simulink model "text"  (R2022a)
settings: Solver=FixedStepAuto  StartTime=0.0  StopTime=10.0  FixedStep=1e-3  RelTol=1e-3  EnableMultiTasking=on
undefined symbols (not defined in the file): A0, A1, D0, D1, PTB2, PTB3, PTC16, PTC17
libraries: etargetslib x16, frdmk64flib x6
settings Model: ExtModeTrigDuration=5  Creator=12791  LastModifiedBy=12791
settings OptimizationCC: EnhancedBackFolding=on  PassReuseOutputArgsAs=Individual arguments  ZeroExternalMemoryAtStartup=off  ZeroInternalMemoryAtStartup=off  MaxStackSize=64  OptimizeBlockOrder=speed  DifferentSizesBufferReuse=on  OptimizationCustomize=off  EfficientTunableParamExpr=on
settings DebuggingCC: ParameterTunabilityLossMsg=error
settings HardwareCC: ProdBitPerPointer=32  ProdBitPerSizeT=32  ProdBitPerPtrDiffT=32  ProdLargestAtomicInteger=Long  ProdLargestAtomicFloat=Double  ProdWordSize=32  ProdHWDeviceType=ARM Compatible->ARM Cortex
settings SFSimCC: MATLABDynamicMemAlloc=off
settings RTWCC: SystemTargetFile=ert.tlc  HardwareBoard=NXP FRDM-K64F  TLCOptions="-aInlineSetEventsForThisBaseRateFcn=TLC_FALSE -aSuppressMultiTaskScheduler=TLC_FALSE  -aRateBasedStepFcn=0"  TemplateMakefile=ert_default_tmf  Toolchain=GNU Tools for ARM Embedded Processors
settings CodeAppCC: ForceParamTrailComments=on  IgnoreCustomStorageClasses=off  OperatorAnnotations=on  SimulinkDataObjDesc=on  SFDataObjDesc=on  InsertBlockDesc=on
settings ERTTargetCC: ExtModeTransport=4  ExtModeMexFile=sendToCommService

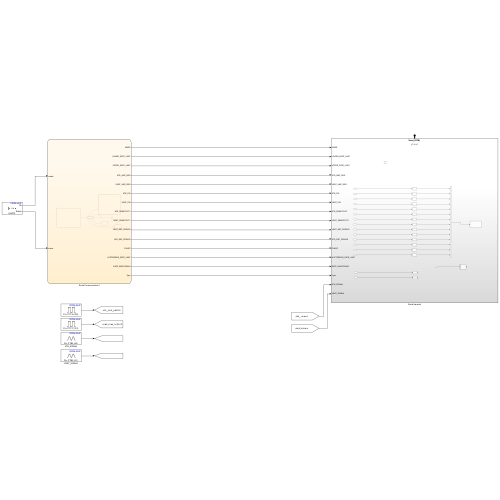
[thumbnail: Simulink's stored preview of the top-level diagram]
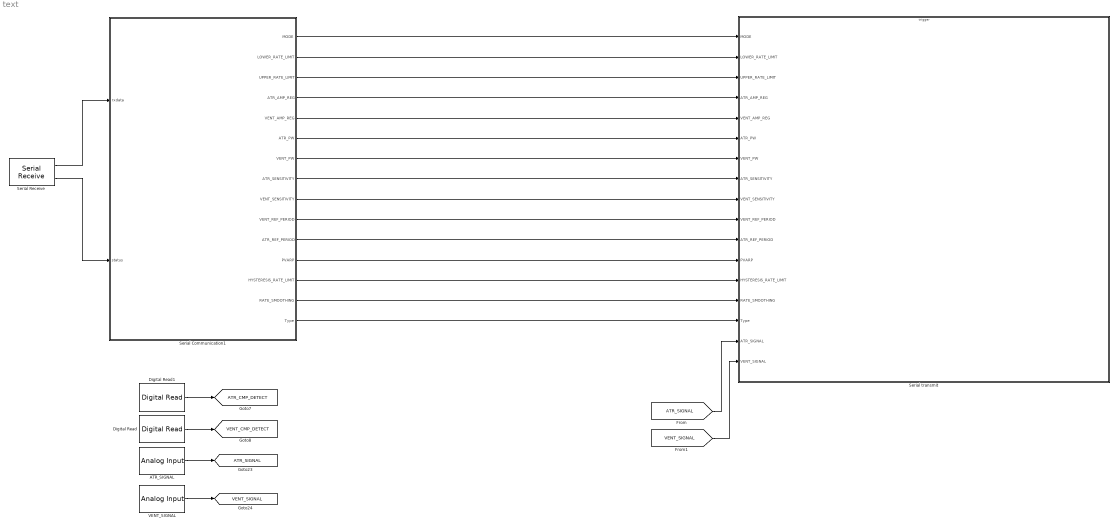
== system text ==
  ATR_SIGNAL : frdmk64flib/Analog Input  Whichpin=PTB2 (A0)  SampleTime=-1
  Digital Read : frdmk64flib/Digital Read  Whichpin=PTC17 (D1)  SampleTime=-1
  Digital Read1 : frdmk64flib/Digital Read  Whichpin=PTC16 (D0)  SampleTime=-1
  Serial Communication1 : Stateflow chart  TreatAsAtomicUnit=on
      settings: PortSchema="{\"entries\":[{\"content\":{\"sides\":[{\"content\":{\"connectorIds\":[\"In1\",\"In2\"]},\"type\":\"ConnectorPlacement.EquallySpacedRectSide\",\"uuid\":\"901574a5-7e09-4852-8827-baac8e876273\"},{\"content\":{\"connectorIds\":[\"Out1\",\"Out2\",\"Out3\",\"Out4\",\"Out12\",\"Out5\",\"Out13\",\"Out14\",\"Out10\",\"Out6\",\"Out11\",\"Out7\",\"Out9\",\"Out8\",\"Out15\"],\"side\":\"RIGHT\"},\"type\":\"ConnectorPlacement.EquallySpacedRectSide\",\"uuid\":\"89d36c37-e833-4dfe-ae0b-2d9eccbce05b\"},{\"content\":{\"connectorIds\":[],\"side\":\"TOP\"},\"type\":\"ConnectorPlacement.EquallySpacedRectSide\",\"uuid\":\"eeb52db1-ccd5-49db-acea-74a4d3271ab8\"}]},\"type\":\"ConnectorPlacement.EquallySpacedConnector\",\"uuid\":\"16ccc146-147c-46a9-b907-deab62e4a6a6\"}],\"packageUris\":[\"http://schema.mathworks.com/mf0/Connector/R2020b\"],\"version\":\"1.0\"}"
  Serial Receive : frdmk64flib/Serial Receive  SCIModule=0  Baudrate=uint32(9600)  Parity=None  StopBits=1  HardwareFlowControl=None  ByteOrder=LittleEndian  DataType=uint8  DataLength=66  BlockingMode=off  OutputStatus=on  SampleTime=-1
  Serial transmit : Subsystem  TreatAsAtomicUnit=on
  VENT_SIGNAL : frdmk64flib/Analog Input  Whichpin=PTB3 (A1)  SampleTime=-1
  tag scope: ATR_CMP_DETECT=global, ATR_SIGNAL=global, VENT_CMP_DETECT=global, VENT_SIGNAL=global
  wires:
  Serial Communication1/1(MODE) -> Serial transmit/1(MODE)
  Serial Communication1/2(LOWER_RATE_LIMIT) -> Serial transmit/2(LOWER_RATE_LIMIT)
  Serial Communication1/3(UPPER_RATE_LIMIT) -> Serial transmit/3(UPPER_RATE_LIMIT)
  Serial Communication1/5(ATR_PW) -> Serial transmit/6(ATR_PW)
  Serial Communication1/13(VENT_PW) -> Serial transmit/7(VENT_PW)
  Serial Communication1/14(ATR_SENSITIVITY) -> Serial transmit/8(ATR_SENSITIVITY)
  Serial Communication1/10(VENT_SENSITIVITY) -> Serial transmit/9(VENT_SENSITIVITY)
  Serial Communication1/7(PVARP) -> Serial transmit/12(PVARP)
  Serial Communication1/9(HYSTERESIS_RATE_LIMIT) -> Serial transmit/13(HYSTERESIS_RATE_LIMIT)
  Serial Communication1/8(RATE_SMOOTHING) -> Serial transmit/14(RATE_SMOOTHING)
  Digital Read1/1 -> [ATR_CMP_DETECT]
  Digital Read/1 -> [VENT_CMP_DETECT]
  Serial Communication1/12(VENT_AMP_REG) -> Serial transmit/5(VENT_AMP_REG)
  Serial Communication1/4(ATR_AMP_REG) -> Serial transmit/4(ATR_AMP_REG)
  ATR_SIGNAL/1 -> [ATR_SIGNAL]
  VENT_SIGNAL/1 -> [VENT_SIGNAL]
  Serial Receive/2 -> Serial Communication1/2(status)
  Serial Receive/1 -> Serial Communication1/1(rxdata)
  Serial Communication1/6(VENT_REF_PERIOD) -> Serial transmit/10(VENT_REF_PERIOD)
  Serial Communication1/11(ATR_REF_PERIOD) -> Serial transmit/11(ATR_REF_PERIOD)
  [VENT_SIGNAL] -> Serial transmit/17(VENT_SIGNAL)
  [ATR_SIGNAL] -> Serial transmit/16(ATR_SIGNAL)
  Serial Communication1/15(Type) -> Serial transmit/15(Type)

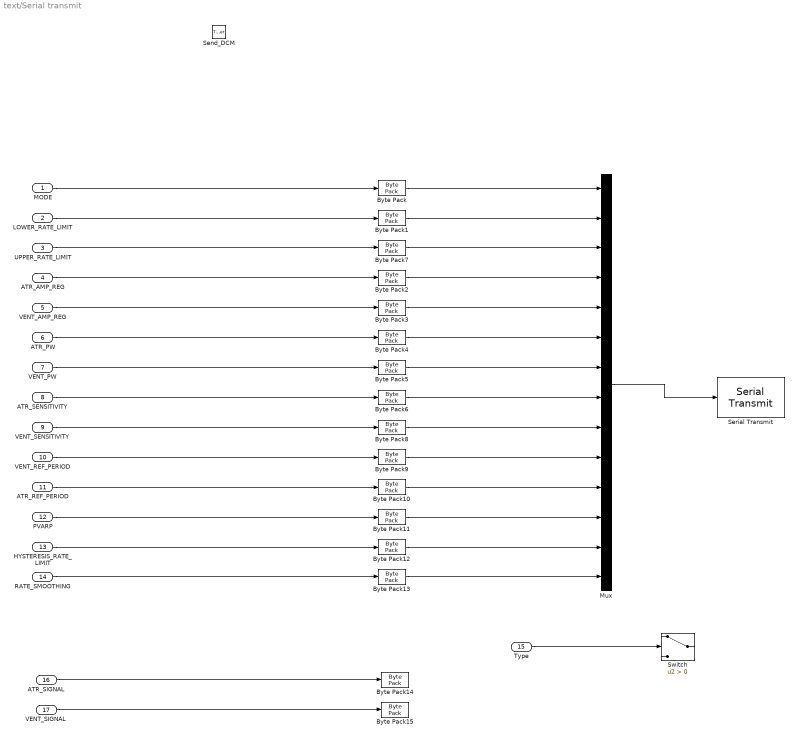
== system text/Serial transmit ==
  MODE : Inport
  LOWER_RATE_LIMIT : Inport  Port=2
  UPPER_RATE_LIMIT : Inport  Port=3
  ATR_AMP_REG : Inport  Port=4
  VENT_AMP_REG : Inport  Port=5
  ATR_PW : Inport  Port=6
  VENT_PW : Inport  Port=7
  ATR_SENSITIVITY : Inport  Port=8
  VENT_SENSITIVITY : Inport  Port=9
  VENT_REF_PERIOD : Inport  Port=10
  ATR_REF_PERIOD : Inport  Port=11
  PVARP : Inport  Port=12
  HYSTERESIS_RATE_LIMIT : Inport  Port=13
  RATE_SMOOTHING : Inport  Port=14
  Type : Inport  Port=15
  ATR_SIGNAL : Inport  Port=16
  VENT_SIGNAL : Inport  Port=17
  Send_DCM : TriggerPort  TriggerType=function-call  IsSimulinkFunction=on  FunctionName=Send_DCM  VariantControl=Variant
  Byte Pack{,1,7,9..13} (8 alike) : etargetslib/Byte Pack  datatypes={'uint16'}  byteAlign=1
  Byte Pack{2..6,8,14..15} (8 alike) : etargetslib/Byte Pack  datatypes={'double'}  byteAlign=1
  Mux : Mux  Inputs=14
  Serial Transmit : frdmk64flib/Serial Transmit  SCIModule=0  Baudrate=uint32(9600)  Parity=None  StopBits=1  HardwareFlowControl=None  ByteOrder=LittleEndian  BlockingMode=on  OutputStatus=off
  Switch : Switch  Criteria=u2 > Threshold  SaturateOnIntegerOverflow=off  InputSameDT=off
  wires:
  MODE/1 -> Byte Pack/1
  LOWER_RATE_LIMIT/1 -> Byte Pack1/1
  UPPER_RATE_LIMIT/1 -> Byte Pack7/1
  ATR_AMP_REG/1 -> Byte Pack2/1
  VENT_AMP_REG/1 -> Byte Pack3/1
  ATR_PW/1 -> Byte Pack4/1
  VENT_PW/1 -> Byte Pack5/1
  VENT_SENSITIVITY/1 -> Byte Pack8/1
  ATR_SENSITIVITY/1 -> Byte Pack6/1
  RATE_SMOOTHING/1 -> Byte Pack13/1
  HYSTERESIS_RATE_LIMIT/1 -> Byte Pack12/1
  PVARP/1 -> Byte Pack11/1
  ATR_REF_PERIOD/1 -> Byte Pack10/1
  VENT_REF_PERIOD/1 -> Byte Pack9/1
  Byte Pack1/1 -> Mux/2
  Byte Pack7/1 -> Mux/3
  Byte Pack/1 -> Mux/1
  Byte Pack2/1 -> Mux/4
  Byte Pack3/1 -> Mux/5
  Byte Pack4/1 -> Mux/6
  Byte Pack5/1 -> Mux/7
  Byte Pack6/1 -> Mux/8
  Byte Pack8/1 -> Mux/9
  Byte Pack9/1 -> Mux/10
  Byte Pack10/1 -> Mux/11
  Byte Pack11/1 -> Mux/12
  Byte Pack12/1 -> Mux/13
  Byte Pack13/1 -> Mux/14
  VENT_SIGNAL/1 -> Byte Pack15/1
  ATR_SIGNAL/1 -> Byte Pack14/1
  Type/1 -> Switch/2
  Mux/1 -> Serial Transmit/1

== stateflow chart text/Serial Communication1 ==
  state SettingParameters
    entry:
    MODE = typecast(rxdata(3:4), 'uint16');
    LOWER_RATE_LIMIT = typecast(rxdata(5:6), 'uint16'); % ppm
    UPPER_RATE_LIMIT = typecast(rxdata(7:8), 'uint16'); % ppm
    ATR_AMP_REG =  typecast(rxdata(9:16), 'double'); % V
    VENT_AMP_REG = typecast(rxdata(17:24), 'double'); % V
    ATR_PW = typecast(rxdata(25:32), 'double'); % ms
    VENT_PW = typecast(rxdata(33:40), 'double'); % ms
    ATR_SENSITIVITY = typecast(rxdata(41:48), 'double'); % mV
    VENT_SENSITIVITY = typecast(rxdata(49:56), 'double'); % mV
    ATR_REF_PERIOD = typecast(rxdata(57:58), 'uint16'); % ms
    VENT_REF_PERIOD = typecast(rxdata(59:60), 'uint16'); % ms
    PVARP = typecast(rxdata(61:62), 'uint16'); % ms
    HYSTERESIS_RATE_LIMIT = typecast(rxdata(63:64), 'uint16'); % ms
    RATE_SMOOTHING = typecast(rxdata(65:66), 'uint16'); % percentage
  state Init
    entry:
    MODE = 2;
    LOWER_RATE_LIMIT = 60;
    UPPER_RATE_LIMIT = 120;
    %MAX_SENSOR_RATE = typecast(rxdata(7:8), 'uint16'); % ppm
    %FIXED_AV_DELAY = typecast(rxdata(9:10), 'uint16'); % ms
    %DYNAMIC_AV_DELAY = rxdata(11); % boolean
    %MIN_DYNAMIC_AV_DELAY =  typecast(rxdata(12:13), 'uint16'); % ms
    %SENSED_AV_DELAY_OFFSET = typecast(rxdata(14:15), 'uint16'); % ms
    ATR_AMP_REG =  3.5; % V
    VENT_AMP_REG = 3.5; % V
    %ATR_AMP_UNREG = typecast(rxdata(9:16), 'double'); % V
    %VENT_AMP_UNREG = typecast(rxdata(9:16), 'double'); % V
    ATR_PW = 0.4; % ms
    VENT_PW = 0.4; % ms
    ATR_SENSITIVITY = 0.75; % mV
    VENT_SENSITIVITY = 2.5; % mV
    ATR_REF_PERIOD = 250; % ms
    VENT_REF_PERIOD = 320; % ms
    PVARP = 250; % ms
    %PVARP_EXTENSION = typecast(rxdata(14:15), 'uint16'); % ms
    HYSTERESIS_RATE_LIMIT = 0; % ms
    RATE_SMOOTHING = 0; % percentage
  state STANDBY
    %Waiting for COM
  state ECHO_PARAM1
    entry:
    Type = 0
    Send_DCM();
  state ECHO_PARAM
    entry:
    Type = 1
    Send_DCM();
  (default) -> Init
  SettingParameters -> STANDBY
  (junction 96) -> STANDBY [order 2]
  (junction 94) -> SettingParameters [order 1] : [rxdata(2) == hex2dec('55')]
  STANDBY -> (junction 96) : [status == 0]
  (junction 96) -> (junction 94) [order 1] : [rxdata(1) == hex2dec('16')]
  Init -> STANDBY
  (junction 94) -> ECHO_PARAM [order 2] : [rxdata(2) == hex2dec('22')]
  (junction 94) -> ECHO_PARAM1 [order 3] : [rxdata(2) == hex2dec('33')]
  ECHO_PARAM -> STANDBY
  ECHO_PARAM1 -> STANDBY
  data: MODE output uint16; LOWER_RATE_LIMIT output uint16; UPPER_RATE_LIMIT output uint16; ATR_AMP_REG output double; ATR_PW output double; rxdata input uint8; status input uint8; VENT_REF_PERIOD output uint16; PVARP output uint16; RATE_SMOOTHING output uint16; HYSTERESIS_RATE_LIMIT output uint16; VENT_SENSITIVITY output double; ATR_REF_PERIOD output uint16; VENT_AMP_REG output double; VENT_PW output double; ATR_SENSITIVITY output; Type output
